simulink model "example1_model"  (R2020a)
settings: Solver=VariableStepAuto  StartTime=0.0  StopTime=40  MaxStep=0.01  RelTol=1e-4  EnableMultiTasking=on
values from neighbouring files (symbols this model uses):
  A = [0 1; -1 0]    [example1.m]
  A1 = [0 0; 0 0]    [example1.m]
  B = [0; 0]    [example1.m]
  B1 = [0; 0]    [example1.m]
  C = [1 0; 0 1]    [example1.m]
  D = [0; 0]    [example1.m]
  DL = [D zeros(2)]    [example1.m]
  L = zeros(2)    [example1.m]
  x0 = 10*x0    [example1.m]
  x0_1 = 1.2 * x0    [example1.m]
libraries: cstblocks x4, simulink x2
settings Model: Creator=amon  LastModifiedBy=amon
settings DataIOCC: LimitDataPoints=on  SaveOutput=off  SaveTime=off
settings OptimizationCC: ExpressionDepthLimit=2147483647  LifeSpan=1
settings DebuggingCC: UnderspecifiedInitializationDetection=Classic  MergeDetectMultiDrivingBlocksExec=none  FcnCallInpInsideContextMsg=warning  AllowSymbolicDim=off  StateNameClashWarn=warning  SFUnexpectedBacktrackingDiag=warning  SFNoUnconditionalDefaultTransitionDiag=warning  SFExecutionAtInitializationDiag=none  ArithmeticOperatorsInVariantConditions=warning
settings SFSimCC: SimUseLocalCustomCode=off  CustomCodeUndefinedFunction=UseInterfaceOnly
settings RTWCC: RTWUseLocalCustomCode=off
settings CodeAppCC: StateflowObjectComments=on
settings GRTTargetCC: TargetLangStandard=C89/C90 (ANSI)  CombineOutputUpdateFcns=off  GRTInterface=on

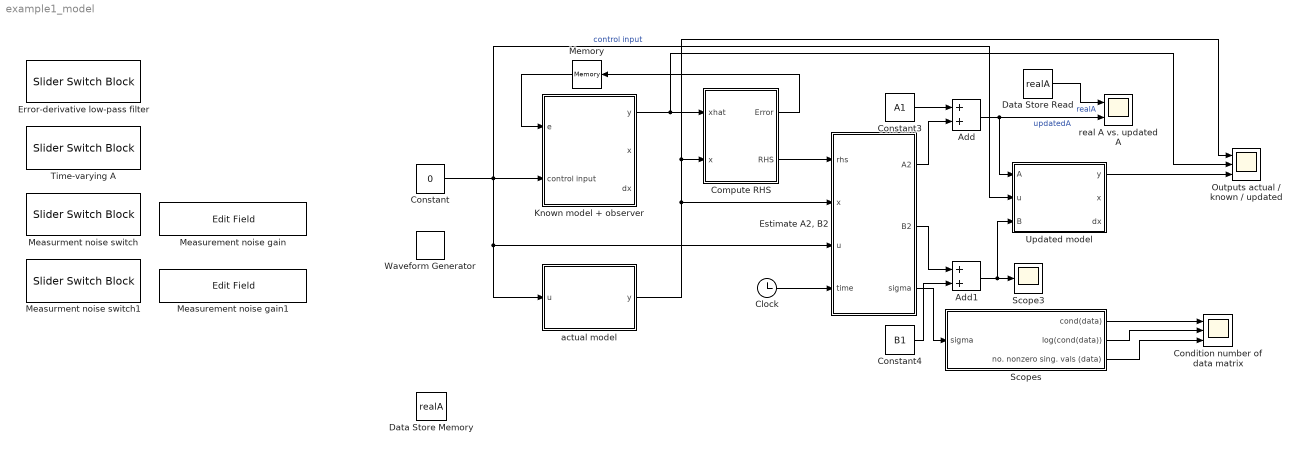
== system example1_model ==
  Add : Sum
  Add1 : Sum
  Clock : Clock
  Compute RHS : Subsystem  mask{A1=A1, L=L, C=C}
  Condition number of data matrix : Scope  NumInputPorts=3
  Constant : Constant  Value=0
  Constant3 : Constant  Value=A1
  Constant4 : Constant  Value=B1
  Data Store Memory : DataStoreMemory  DataStoreName=realA  ReadBeforeWriteMsg=warning  WriteAfterWriteMsg=warning  WriteAfterReadMsg=warning  InitialValue=A  ShowAdditionalParam=off
  Data Store Read : DataStoreRead  DataStoreName=realA
  Error-derivative low-pass filter : SliderSwitchBlock
      settings: Values={{'Off', 'On'}, [0 1]}
  "Estimate A2, B2" : MATLAB Function  TreatAsAtomicUnit=on
  Known model + observer : Subsystem  mask{A=A1, B=B1, C=C, D=DL, L=L, x0=x0_1}
  Measurement noise gain : EditField  LabelPosition=Hide  ShowInitialText=on  Alignment=Center
  Measurement noise gain1 : EditField  LabelPosition=Hide  ShowInitialText=on  Alignment=Center
  Measurment noise switch : SliderSwitchBlock
      settings: Values={{'Off', 'On'}, [0 1]}
  Measurment noise switch1 : SliderSwitchBlock
      settings: Values={{'Off', 'On'}, [0 1]}
  Memory : Memory
  Outputs actual / known / updated : Scope  NumInputPorts=3
  Scope3 : Scope
  Scopes : Subsystem
  Time-varying A : SliderSwitchBlock
      settings: Values={{'Off', 'On'}, [0 1]}
  Updated model : Subsystem  mask{C=C, D=D, x0=x0}
  Waveform Generator : simulink/Sources/Waveform Generator  OutMin=[]  OutMax=[]  OutDataTypeStr=double  SelectedSignal=1  Signals=sin('Amplitude', 10, 'Frequency', 3, 'Phase', 1)  BlockNames=MultiportSwitch_c76754861baa43b  SampleTime=0.1
  actual model : Subsystem  mask{A=A, B=B, C=C, D=D, Knoise=0.1, x0=x0}
      mask prompts: Knoise "Noise gain"
  real A vs. updated A : Scope  NumInputPorts=2
  wires:
  Add1/1 -> Scope3/1, Updated model/3(B)
  Constant3/1 -> Add/1
  Add/1 -> Updated model/1(A), real A vs. updated A/2  "updatedA"
  "Estimate A2, B2"/2(B2) -> Add1/1
  Compute RHS/2(RHS) -> "Estimate A2, B2"/1(rhs)
  "Estimate A2, B2"/1(A2) -> Add/2
  Compute RHS/1(Error) -> Memory/1
  actual model/1(y) -> Outputs actual / known / updated/1, Compute RHS/2(x), "Estimate A2, B2"/2(x)
  Constant4/1 -> Add1/2
  Clock/1 -> "Estimate A2, B2"/4(time)
  Known model + observer/1(y) -> Compute RHS/1(xhat), Outputs actual / known / updated/2
  Constant/1 -> "Estimate A2, B2"/3(u), actual model/1(u), Updated model/2(u), Known model + observer/2(control input)  "control input"
  Memory/1 -> Known model + observer/1(e)
  "Estimate A2, B2"/3(sigma) -> Scopes/1(sigma)
  Updated model/1(y) -> Outputs actual / known / updated/3
  Data Store Read/1 -> real A vs. updated A/1  "realA"
  Scopes/1(cond(data)) -> Condition number of data matrix/1
  Scopes/2(log(cond(data))) -> Condition number of data matrix/2
  Scopes/3(no. nonzero sing. vals (data)) -> Condition number of data matrix/3

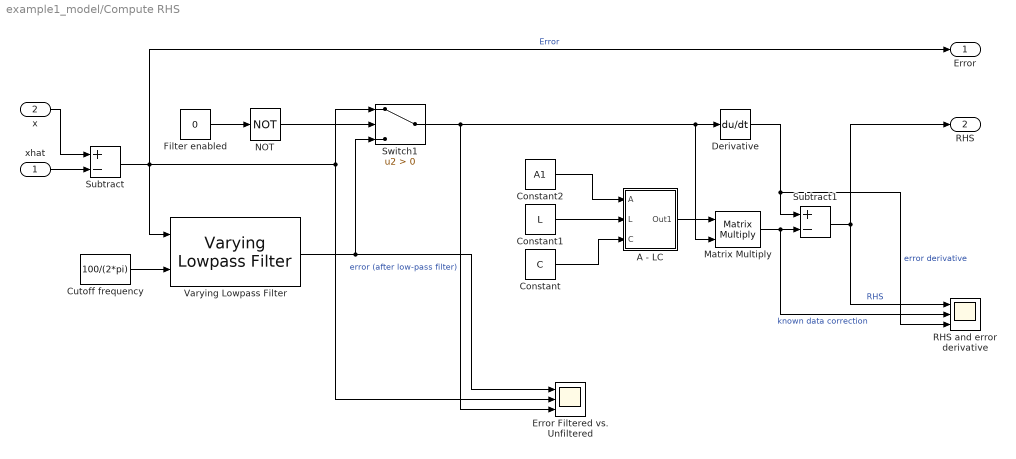
== system example1_model/Compute RHS ==
  xhat : Inport
  x : Inport  Port=2
  A - LC : Subsystem
  Constant : Constant  Value=C
  Constant1 : Constant  Value=L
  Constant2 : Constant  Value=A1
  Cutoff frequency : Constant  Value=100/(2*pi)  SampleTime=0.01
  Derivative : Derivative
  Error Filtered vs. Unfiltered : Scope  NumInputPorts=3
  Filter enabled : Constant  Value=0
  Matrix Multiply : Product  Multiplication=Matrix(*)
  NOT : Logic  Operator=NOT  IconShape=distinctive  AllPortsSameDT=off  OutDataTypeStr=boolean
  RHS and error derivative : Scope  NumInputPorts=3
  Subtract : Sum  Inputs=+-
  Subtract1 : Sum  Inputs=+-
  Switch1 : Switch  Criteria=u2 > Threshold
  Varying Lowpass Filter : cstblocks/Linear Parameter Varying/Varying Lowpass Filter  N=1
  Error : Outport
  RHS : Outport  Port=2
  wires:
  Subtract/1 -> Error Filtered vs. Unfiltered/2, Switch1/1, Varying Lowpass Filter/1, Error/1  "Error"
  Varying Lowpass Filter/1 -> Error Filtered vs. Unfiltered/1, Switch1/3
  Constant/1 -> A - LC/3(C)
  Filter enabled/1 -> NOT/1
  Constant2/1 -> A - LC/1(A)
  A - LC/1(Out1) -> Matrix Multiply/1
  Subtract1/1 -> RHS/1, RHS and error derivative/1  "RHS"
  xhat/1 -> Subtract/2
  Switch1/1 -> Matrix Multiply/2, Derivative/1, Error Filtered vs. Unfiltered/3  "error (after low-pass filter)"
  Cutoff frequency/1 -> Varying Lowpass Filter/2
  x/1 -> Subtract/1
  Matrix Multiply/1 -> RHS and error derivative/2, Subtract1/2  "known data correction"
  Derivative/1 -> RHS and error derivative/3, Subtract1/1  "error derivative"
  NOT/1 -> Switch1/2
  Constant1/1 -> A - LC/2(L)

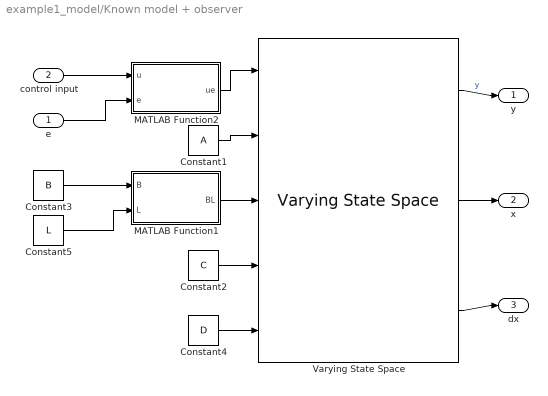
== system example1_model/Known model + observer ==
  e : Inport
  control input : Inport  Port=2
  Constant1 : Constant  Value=A
  Constant2 : Constant  Value=C
  Constant3 : Constant  Value=B
  Constant4 : Constant  Value=D
  Constant5 : Constant  Value=L
  MATLAB Function1 : MATLAB Function  TreatAsAtomicUnit=on
  MATLAB Function2 : MATLAB Function  TreatAsAtomicUnit=on
  Varying State Space : cstblocks/Linear Parameter Varying/Varying State Space  x0=x0  xNames=''  OutputX=on  OutputDX=on
  y : Outport
  x : Outport  Port=2
  dx : Outport  Port=3
  wires:
  Constant1/1 -> Varying State Space/2
  Varying State Space/2 -> x/1
  Constant4/1 -> Varying State Space/5
  Varying State Space/3 -> dx/1
  control input/1 -> MATLAB Function2/1(u)
  Constant2/1 -> Varying State Space/4
  e/1 -> MATLAB Function2/2(e)
  Varying State Space/1 -> y/1  "y"
  Constant3/1 -> MATLAB Function1/1(B)
  MATLAB Function2/1(ue) -> Varying State Space/1
  MATLAB Function1/1(BL) -> Varying State Space/3
  Constant5/1 -> MATLAB Function1/2(L)

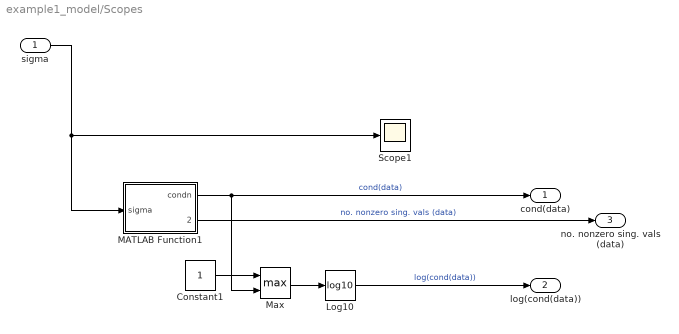
== system example1_model/Scopes ==
  sigma : Inport
  Constant1 : Constant
  Log10 : Math  Operator=log10  SaturateOnIntegerOverflow=on
  MATLAB Function1 : MATLAB Function  TreatAsAtomicUnit=on
  Max : MinMax  Function=max  Inputs=2
  Scope1 : Scope
  cond(data) : Outport
  log(cond(data)) : Outport  Port=2
  no. nonzero sing. vals (data) : Outport  Port=3
  wires:
  sigma/1 -> MATLAB Function1/1(sigma), Scope1/1
  Log10/1 -> log(cond(data))/1  "log(cond(data))"
  Max/1 -> Log10/1
  MATLAB Function1/1(condn) -> cond(data)/1, Max/2  "cond(data)"
  Constant1/1 -> Max/1
  MATLAB Function1/2(n_nzsigma) -> no. nonzero sing. vals (data)/1  "no. nonzero sing. vals (data)"

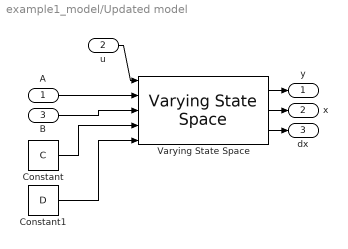
== system example1_model/Updated model ==
  A : Inport
  u : Inport  Port=2
  B : Inport  Port=3
  Constant : Constant  Value=C
  Constant1 : Constant  Value=D
  Varying State Space : cstblocks/Linear Parameter Varying/Varying State Space  x0=x0  xNames=''  OutputX=on  OutputDX=on
  y : Outport
  x : Outport  Port=2
  dx : Outport  Port=3
  wires:
  Constant1/1 -> Varying State Space/5
  Varying State Space/2 -> x/1
  Constant/1 -> Varying State Space/4
  u/1 -> Varying State Space/1
  Varying State Space/1 -> y/1
  Varying State Space/3 -> dx/1
  A/1 -> Varying State Space/2
  B/1 -> Varying State Space/3

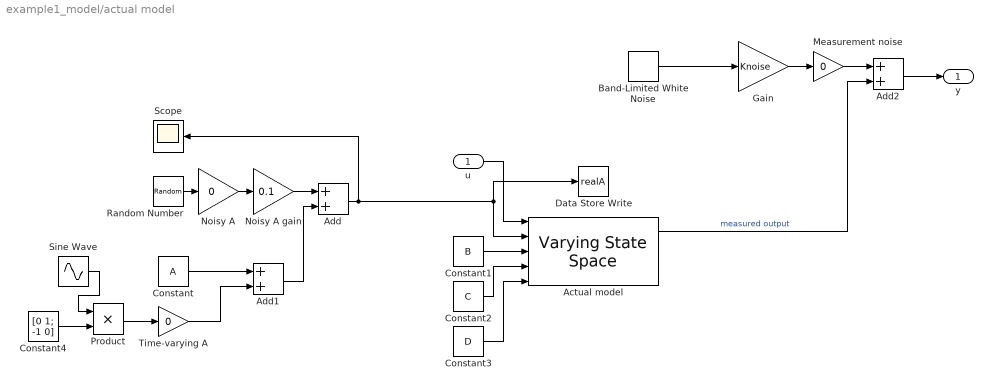
== system example1_model/actual model ==
  u : Inport
  Actual model : cstblocks/Linear Parameter Varying/Varying State Space  x0=x0  xNames=''  OutputX=on  OutputDX=on
  Add : Sum
  Add1 : Sum
  Add2 : Sum
  Band-Limited White Noise : simulink/Sources/Band-Limited White Noise  Cov=[0.001; 0.001]  Ts=0.01  seed=[23341]
  Constant : Constant  Value=A
  Constant1 : Constant  Value=B
  Constant2 : Constant  Value=C
  Constant3 : Constant  Value=D
  Constant4 : Constant  Value=[0 1; -1 0]
  Data Store Write : DataStoreWrite  DataStoreName=realA
  Gain : Gain  Gain=Knoise
  Measurement noise : Gain  Gain=0
  Noisy A : Gain  Gain=0
  Noisy A gain : Gain  Gain=0.1
  Product : Product
  Random Number : RandomNumber  Mean=[1 1; 1 1]  Variance=0.1  SampleTime=0.1
  Scope : Scope
  Sine Wave : Sin  Frequency=0.05*(2*pi)  SampleTime=0
  Time-varying A : Gain  Gain=0
  y : Outport
  wires:
  Add2/1 -> y/1
  Actual model/1 -> Add2/2  "measured output"
  Gain/1 -> Measurement noise/1
  u/1 -> Actual model/1
  Band-Limited White Noise/1 -> Gain/1
  Constant1/1 -> Actual model/3
  Constant3/1 -> Actual model/5
  Constant2/1 -> Actual model/4
  Constant/1 -> Add1/1
  Random Number/1 -> Noisy A/1
  Noisy A/1 -> Noisy A gain/1
  Add/1 -> Scope/1, Actual model/2, Data Store Write/1
  Sine Wave/1 -> Product/1
  Product/1 -> Time-varying A/1
  Constant4/1 -> Product/2
  Add1/1 -> Add/2
  Time-varying A/1 -> Add1/2
  Measurement noise/1 -> Add2/1
  Noisy A gain/1 -> Add/1

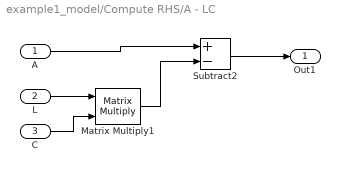
== system example1_model/Compute RHS/A - LC ==
  A : Inport
  L : Inport  Port=2
  C : Inport  Port=3
  Matrix Multiply1 : Product  Multiplication=Matrix(*)
  Subtract2 : Sum  Inputs=+-
  Out1 : Outport
  wires:
  Subtract2/1 -> Out1/1
  A/1 -> Subtract2/1
  Matrix Multiply1/1 -> Subtract2/2
  L/1 -> Matrix Multiply1/1
  C/1 -> Matrix Multiply1/2

== matlab function example1_model/Known model + observer/MATLAB Function1 ==
  data: B input; BL output; L input
function BL = append_hori(B,L)
BL = [B L];

== matlab function example1_model/Estimate A2, B2 ==
  settings: updateMethod=DISCRETE
  data: rhs input; x input; u input; A2 output; time input; B2 output; sigma output size=3
function [A2, B2, sigma] = fcn(rhs, x, u, time)

persistent rhs_store u_store x_store 
persistent time_last store_index
persistent time_debug_last

dt_debug = 1; % can be used to stop simulation at certain time
dt_min = 0.01; % time between new data points
store_maxsize = 50; % number of data points used for estimation

% initialize persistent variables
if isempty(store_index)
    store_index = 0;
    rhs_store = nan(size(rhs,1),store_maxsize);
    x_store = nan(size(x,1),store_maxsize);
    u_store = nan(size(u,1),store_maxsize);
end
if isempty(time_last)
    time_last = time;
    time_debug_last = time;
    A2 = zeros(size(rhs,1));
    B2 = zeros(size(rhs,1), size(u,1));
    sigma = zeros(size(rhs,1) + size(u,1),1);
    return
end

% store a new data point every dt_min seconds
if time - time_last >= dt_min
    time_last = time;
    if store_index < store_maxsize
        store_index = store_index + 1;
        rhs_store(:,store_index) = rhs;
        x_store(:,store_index) = x;
        u_store(:,store_index) = u;
    else
        rhs_store = [rhs_store(:,2:end) rhs];
        x_store = [x_store(:,2:end) x];
        u_store = [u_store(:,2:end) u];
    end
end

% place debugging point here to stop simulation at specified time
if time - time_debug_last >= dt_debug && time > 28
    time_debug_last = time;
end

sigma = zeros(size(rhs,1) + size(u,1),1);
if store_index >= 1
    % compute SVD of data points
    [U,S,V] = svd([x_store(:,1:store_index); u_store(:,1:store_index)], 'econ');
    % filter out singular values that are close to zero
    nz_log = (S(1,1) ./ diag(S)) < 1/(100*eps);
    S = diag(S(diag(nz_log)));
    U = U(:,nz_log);
    V = V(:,nz_log);
    % invert the nonsingular part that is left after truncation
    A2B2 = rhs_store(:,1:store_index) * V * (S \ U');
    % split output into A2 and B2
    A2 = A2B2(:,1:size(rhs,1));
    B2 = A2B2(:,size(rhs,1)+1);
    sigma(1:sum(nz_log)) = diag(S);
else
    A2 = zeros(size(rhs,1));
    B2 = zeros(size(rhs,1), size(u,1));
end

== matlab function example1_model/Scopes/MATLAB Function1 ==
  data: sigma input; condn output; n_nzsigma output
function [condn, n_nzsigma] = fcn(sigma)
is_sigma_nz = sigma > 0;
sigma_nz = sigma(is_sigma_nz);
n_nzsigma = sum(is_sigma_nz);
if ~isempty(sigma_nz)
    condn = max(sigma_nz) / min(sigma_nz);
else
    condn = -1;
end

== matlab function example1_model/Known model + observer/MATLAB Function2 ==
  data: u input; ue output; e input
function ue = append_vert(u,e)
ue  = [u;e];
